simulink model "quad_SMC"  (R2021a)
settings: Solver=ode3  StartTime=0.0  StopTime=30  FixedStep=0.01  RelTol=1e-3  EnableMultiTasking=on
values from neighbouring files (symbols this model uses):
  g = 9.8    [init_landing.m]
  m = 0.486    [init_landing.m]
undefined symbols (not defined in the file or in its folder): attitude_control, model, position_control, sigbuilder_block, sliding_var
libraries: simulink x7, fuzblock x6, eeGeneralControl x3
settings Model: Creator=smishra  LastModifiedBy=fairu
settings SolverCC: AlgebraicLoopSolver=TrustRegion
settings DataIOCC: LimitDataPoints=on  SaveFormat=Array  ReturnWorkspaceOutputs=off  Refine=5
settings OptimizationCC: LifeSpan=inf
settings DebuggingCC: SFUnexpectedBacktrackingDiag=warning  SFNoUnconditionalDefaultTransitionDiag=warning  SFExecutionAtInitializationDiag=none  SFMachineParentedDataDiag=warning  ArithmeticOperatorsInVariantConditions=warning
settings HardwareCC: ProdBitPerPointer=32  ProdBitPerSizeT=32  ProdBitPerPtrDiffT=32  ProdLargestAtomicFloat=None  ProdIntDivRoundTo=Undefined  ProdEndianess=Unspecified  ProdWordSize=32  ProdHWDeviceType=32-bit Generic
settings ModelReferenceCC: PropagateSignalLabelsOutOfModel=off
settings SFSimCC: SimUseLocalCustomCode=off  CustomCodeUndefinedFunction=UseInterfaceOnly
settings RTWCC: RTWUseLocalCustomCode=off
settings CodeAppCC: StateflowObjectComments=on
settings GRTTargetCC: TargetLangStandard=C89/C90 (ANSI)
settings ConfigComp: CovMetricSettings=dw  CovSaveCumulativeToWorkspaceVar=on  CovSaveSingleToWorkspaceVar=on  CovExternalEMLEnable=off

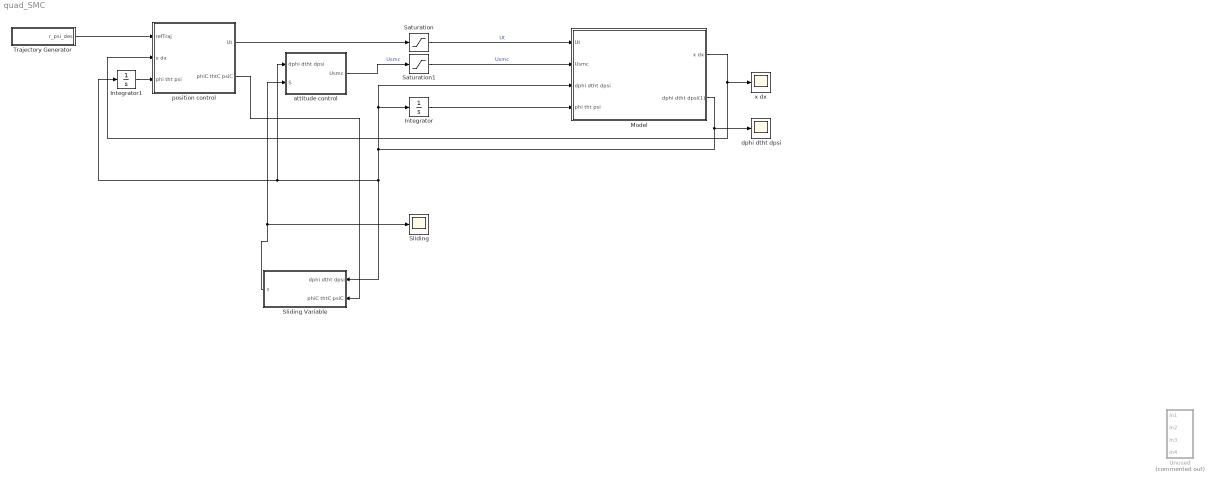
== system quad_SMC ==
  Integrator : Integrator
  Integrator1 : Integrator
  Model : Subsystem
  Saturation : Saturate  UpperLimit=2*m*g  LowerLimit=0
  Saturation1 : Saturate  UpperLimit=0.2  LowerLimit=-0.2
  Sliding : Scope
  Sliding Variable : Subsystem
  Trajectory Generator : Subsystem
  Unused : Subsystem  Commented=on
  attitude control : Subsystem
  dphi dtht dpsi : Scope
  position control : Subsystem
  x dx : Scope
  wires:
  Trajectory Generator/1(r_psi_des) -> position control/1(refTraj)
  Model/2(dphi dtht dpsi(1)) -> dphi dtht dpsi/1, Integrator1/1, attitude control/1(dphi dtht dpsi), Sliding Variable/1(dphi dtht dpsi), Integrator/1, Model/3(dphi dtht dpsi)
  Integrator/1 -> Model/4(phi tht psi)
  Integrator1/1 -> position control/3(phi tht psi)
  Model/1(x dx) -> x dx/1, position control/2(x dx)
  Sliding Variable/1(s) -> attitude control/2(S), Sliding/1
  position control/2(phiC thtC psiC) -> Sliding Variable/2(phiC thtC psiC)
  Saturation/1 -> Model/1(Ut)  "Ut"
  position control/1(Ut) -> Saturation/1
  attitude control/1(Usmc) -> Saturation1/1  "Usmc"
  Saturation1/1 -> Model/2(Usmc)  "Usmc"

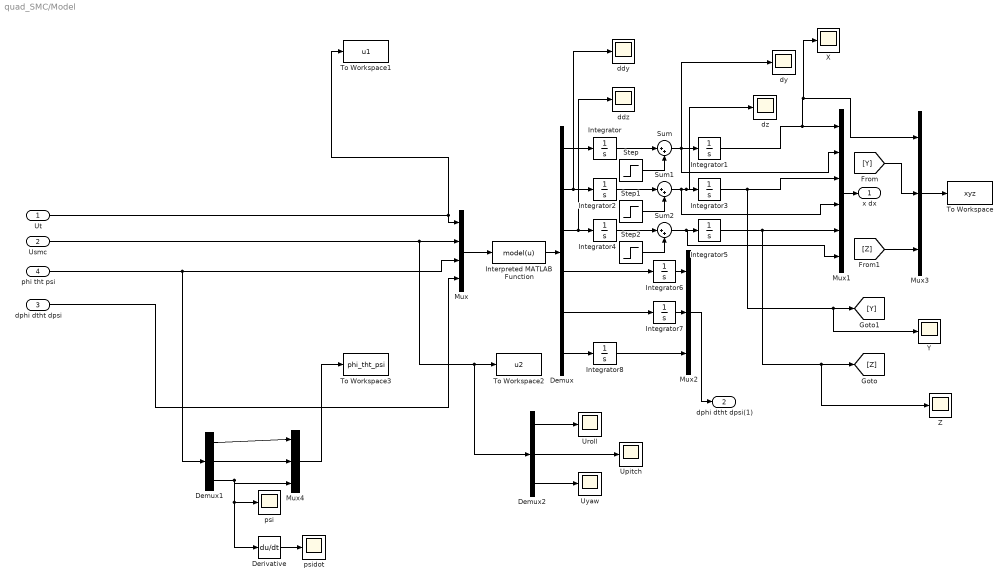
== system quad_SMC/Model ==
  Ut : Inport
  Usmc : Inport  Port=2
  dphi dtht dpsi : Inport  Port=3
  phi tht psi : Inport  Port=4
  Demux : Demux  Outputs=6
  Demux1 : Demux  Outputs=3
  Demux2 : Demux  Outputs=3
  Derivative : Derivative
  Integrator{,1..2,4..8} (8 alike) : Integrator
  Integrator3 : Integrator  InitialCondition=8
  Interpreted MATLAB Function : MATLABFcn  MATLABFcn=model(u)  OutputDimensions=6
  Mux : Mux
  Mux1 : Mux  Inputs=6
  Mux2 : Mux  Inputs=3
  Mux3 : Mux  Inputs=3
  Mux4 : Mux  Inputs=3
  Step : Step  Time=25  After=5  SampleTime=0
  Step1 : Step  Time=25  After=5  SampleTime=0
  Step2 : Step  Time=25  After=5  SampleTime=0
  Sum : Sum  Inputs=|++
  Sum1 : Sum  Inputs=|++
  Sum2 : Sum  Inputs=|++
  To Workspace : ToWorkspace  VariableName=xyz  SampleTime=-1
  To Workspace1 : ToWorkspace  VariableName=u1  SampleTime=-1
  To Workspace2 : ToWorkspace  VariableName=u2  SampleTime=-1
  To Workspace3 : ToWorkspace  VariableName=phi_tht_psi  SampleTime=-1
  Upitch : Scope
  Uroll : Scope
  Uyaw : Scope
  X : Scope
  Y : Scope
  Z : Scope
  ddy : Scope
  ddz : Scope
  dy : Scope
  dz : Scope
  psi : Scope
  psidot : Scope
  x dx : Outport
  dphi dtht dpsi(1) : Outport  Port=2
  wires:
  Mux2/1 -> dphi dtht dpsi(1)/1
  Mux1/1 -> x dx/1
  Mux/1 -> Interpreted MATLAB Function/1
  Integrator3/1 -> Mux1/3, Y/1, [Y]
  Demux/3 -> ddz/1, Integrator4/1
  Demux/1 -> Integrator/1
  Integrator1/1 -> X/1, Mux3/1, Mux1/1
  Integrator7/1 -> Mux2/2
  Interpreted MATLAB Function/1 -> Demux/1
  Integrator8/1 -> Mux2/3
  Demux/2 -> ddy/1, Integrator2/1
  Integrator6/1 -> Mux2/1
  phi tht psi/1 -> Demux1/1, Mux/3
  Mux3/1 -> To Workspace/1
  Ut/1 -> Mux/1, To Workspace1/1
  Usmc/1 -> Mux/2, Demux2/1, To Workspace2/1
  dphi dtht dpsi/1 -> Mux/4
  Demux/4 -> Integrator6/1
  Demux/5 -> Integrator7/1
  Demux/6 -> Integrator8/1
  Integrator/1 -> Sum/1
  Sum/1 -> dy/1, Mux1/2, Integrator1/1
  Integrator2/1 -> Sum1/1
  Sum1/1 -> Mux1/4, dz/1, Integrator3/1
  Integrator4/1 -> Sum2/1
  Step/1 -> Sum/2
  Step1/1 -> Sum1/2
  Step2/1 -> Sum2/2
  Sum2/1 -> Mux1/6, Integrator5/1
  Integrator5/1 -> Z/1, [Z], Mux1/5
  [Y] -> Mux3/2
  [Z] -> Mux3/3
  Demux1/1 -> Mux4/1
  Demux1/2 -> Mux4/2
  Demux1/3 -> Derivative/1, psi/1, Mux4/3
  Mux4/1 -> To Workspace3/1
  Derivative/1 -> psidot/1
  Demux2/1 -> Uroll/1
  Demux2/2 -> Upitch/1
  Demux2/3 -> Uyaw/1

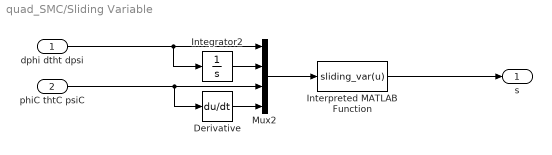
== system quad_SMC/Sliding Variable ==
  dphi dtht dpsi : Inport
  phiC thtC psiC : Inport  Port=2
  Derivative : Derivative
  Integrator2 : Integrator
  Interpreted MATLAB Function : MATLABFcn  MATLABFcn=sliding_var(u)  OutputDimensions=3
  Mux2 : Mux
  s : Outport
  wires:
  Integrator2/1 -> Mux2/2
  Mux2/1 -> Interpreted MATLAB Function/1
  dphi dtht dpsi/1 -> Integrator2/1, Mux2/1
  Interpreted MATLAB Function/1 -> s/1
  phiC thtC psiC/1 -> Derivative/1, Mux2/3
  Derivative/1 -> Mux2/4

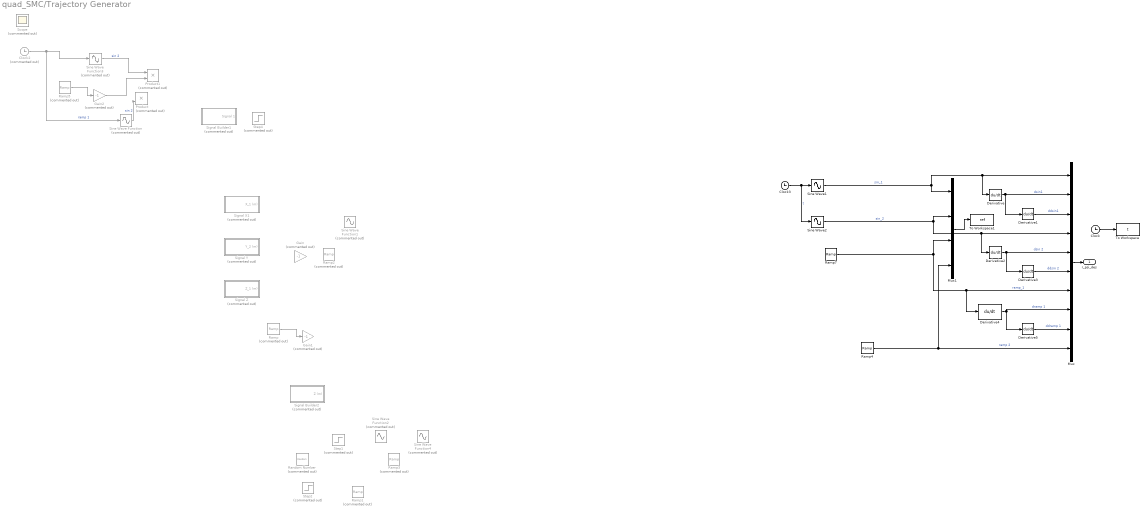
== system quad_SMC/Trajectory Generator ==
  Clock : Clock
  Clock2 : Clock  Commented=on
  Clock3 : Clock
  Derivative{,1..5} (6 alike) : Derivative
  Gain : Gain  Commented=on  Gain=-1
  Gain1 : Gain  Commented=on  Gain=-1
  Gain2 : Gain  Commented=on  Gain=-1
  Mux : Mux  Inputs=10
  Mux1 : Mux
  Product : Product  Commented=on
  Product1 : Product  Commented=on
  Ramp : simulink/Sources/Ramp  Commented=on  slope=1  start=0  InitialOutput=0
  Ramp1 : simulink/Sources/Ramp  Commented=on  slope=0  start=0  InitialOutput=0
  Ramp2 : simulink/Sources/Ramp  Commented=on  slope=0.2  start=0  InitialOutput=-10
  Ramp3 : simulink/Sources/Ramp  Commented=on  slope=0.2  start=0  InitialOutput=-8
  Ramp4 : simulink/Sources/Ramp  slope=0  start=0  InitialOutput=0
  Ramp5 : simulink/Sources/Ramp  Commented=on  slope=1  start=0  InitialOutput=0
  Ramp7 : simulink/Sources/Ramp  slope=0.2  start=0  InitialOutput=0
  Random Number : RandomNumber  Commented=on  SampleTime=0
  Scope : Scope  Commented=on
  Signal Builder1 : Subsystem  Tag=STV Subsys  Commented=on  LoadFcn=sigbuilder_block('load');  StartFcn=sigbuilder_block('start');  StopFcn=sigbuilder_block('stop');  ClipboardFcn=sigbuilder_block('clipboard');  mask(Sigbuilder block){tuvar=[0:10]}
      mask help: Simulink:masks:SigbuilderBlock_MD
      mask init:
      | if ~strcmp(get_param(bdroot(gcbh),'SimulationStatus'),'stopped') tuvar = sigbuilder_block('maskInit'); end
      settings: CopyFcn=sigbuilder_block('copy');  DeleteFcn=sigbuilder_block('delete');  ModelCloseFcn=sigbuilder_block('modelClose');  PreSaveFcn=sigbuilder_block('preSave');  PauseFcn=sigbuilder_block('pause');  ContinueFcn=sigbuilder_block('continue');  NameChangeFcn=sigbuilder_block('namechange');  OpenFcn=sigbuilder_block('open',[411 128.5 543.5 351.5 ]);  CloseFcn=sigbuilder_block('close');
      mask Display: plot(0, 0, 100, 100,[2, 2, 32, 32, 2], [68, 8, 8, 68, 68],[32, 2], [38, 38], [32, 19, 2],[53, 60, 44], [32, 17, 17, 2],[16, 16, 31, 31]);txt = getActiveGroup(gcbh);text(2, 100, txt,'verticalAlignment', 'top');
  Signal Builder2 : Subsystem  Tag=STV Subsys  Commented=on  LoadFcn=sigbuilder_block('load');  StartFcn=sigbuilder_block('start');  StopFcn=sigbuilder_block('stop');  ClipboardFcn=sigbuilder_block('clipboard');  mask(Sigbuilder block){tuvar=[0:10]}
      mask help: Simulink:masks:SigbuilderBlock_MD
      mask init:
      | if ~strcmp(get_param(bdroot(gcbh),'SimulationStatus'),'stopped') tuvar = sigbuilder_block('maskInit'); end
      settings: CopyFcn=sigbuilder_block('copy');  DeleteFcn=sigbuilder_block('delete');  ModelCloseFcn=sigbuilder_block('modelClose');  PreSaveFcn=sigbuilder_block('preSave');  PauseFcn=sigbuilder_block('pause');  ContinueFcn=sigbuilder_block('continue');  NameChangeFcn=sigbuilder_block('namechange');  OpenFcn=sigbuilder_block('open',[5.5 30 949 418 ]);  CloseFcn=sigbuilder_block('close');
      mask Display: plot(0, 0, 100, 100,[2, 2, 32, 32, 2], [68, 8, 8, 68, 68],[32, 2], [38, 38], [32, 19, 2],[53, 60, 44], [32, 17, 17, 2],[16, 16, 31, 31]);txt = getActiveGroup(gcbh);text(2, 100, txt,'verticalAlignment', 'top');
  Signal X1 : Subsystem  Tag=STV Subsys  Commented=on  LoadFcn=sigbuilder_block('load');  StartFcn=sigbuilder_block('start');  StopFcn=sigbuilder_block('stop');  ClipboardFcn=sigbuilder_block('clipboard');  mask(Sigbuilder block){tuvar=[0:10]}
      mask help: Simulink:masks:SigbuilderBlock_MD
      mask init:
      | if ~strcmp(get_param(bdroot(gcbh),'SimulationStatus'),'stopped') tuvar = sigbuilder_block('maskInit'); end
      settings: CopyFcn=sigbuilder_block('copy');  DeleteFcn=sigbuilder_block('delete');  ModelCloseFcn=sigbuilder_block('modelClose');  PreSaveFcn=sigbuilder_block('preSave');  PauseFcn=sigbuilder_block('pause');  ContinueFcn=sigbuilder_block('continue');  NameChangeFcn=sigbuilder_block('namechange');  OpenFcn=sigbuilder_block('open',[411 128.5 543.5 351.5 ]);  CloseFcn=sigbuilder_block('close');
      mask Display: plot(0, 0, 100, 100,[2, 2, 32, 32, 2], [68, 8, 8, 68, 68],[32, 2], [38, 38], [32, 19, 2],[53, 60, 44], [32, 17, 17, 2],[16, 16, 31, 31]);txt = getActiveGroup(gcbh);text(2, 100, txt,'verticalAlignment', 'top');
  Signal Y : Subsystem  Tag=STV Subsys  Commented=on  LoadFcn=sigbuilder_block('load');  StartFcn=sigbuilder_block('start');  StopFcn=sigbuilder_block('stop');  ClipboardFcn=sigbuilder_block('clipboard');  mask(Sigbuilder block){tuvar=[0:10]}
      mask help: Simulink:masks:SigbuilderBlock_MD
      mask init:
      | if ~strcmp(get_param(bdroot(gcbh),'SimulationStatus'),'stopped') tuvar = sigbuilder_block('maskInit'); end
      settings: CopyFcn=sigbuilder_block('copy');  DeleteFcn=sigbuilder_block('delete');  ModelCloseFcn=sigbuilder_block('modelClose');  PreSaveFcn=sigbuilder_block('preSave');  PauseFcn=sigbuilder_block('pause');  ContinueFcn=sigbuilder_block('continue');  NameChangeFcn=sigbuilder_block('namechange');  OpenFcn=sigbuilder_block('open',[411 128.5 543.5 351.5 ]);  CloseFcn=sigbuilder_block('close');
      mask Display: plot(0, 0, 100, 100,[2, 2, 32, 32, 2], [68, 8, 8, 68, 68],[32, 2], [38, 38], [32, 19, 2],[53, 60, 44], [32, 17, 17, 2],[16, 16, 31, 31]);txt = getActiveGroup(gcbh);text(2, 100, txt,'verticalAlignment', 'top');
  Signal Z : Subsystem  Tag=STV Subsys  Commented=on  LoadFcn=sigbuilder_block('load');  StartFcn=sigbuilder_block('start');  StopFcn=sigbuilder_block('stop');  ClipboardFcn=sigbuilder_block('clipboard');  mask(Sigbuilder block){tuvar=[0:10]}
      mask help: Simulink:masks:SigbuilderBlock_MD
      mask init:
      | if ~strcmp(get_param(bdroot(gcbh),'SimulationStatus'),'stopped') tuvar = sigbuilder_block('maskInit'); end
      settings: CopyFcn=sigbuilder_block('copy');  DeleteFcn=sigbuilder_block('delete');  ModelCloseFcn=sigbuilder_block('modelClose');  PreSaveFcn=sigbuilder_block('preSave');  PauseFcn=sigbuilder_block('pause');  ContinueFcn=sigbuilder_block('continue');  NameChangeFcn=sigbuilder_block('namechange');  OpenFcn=sigbuilder_block('open',[411 128.5 543.5 351.5 ]);  CloseFcn=sigbuilder_block('close');
      mask Display: plot(0, 0, 100, 100,[2, 2, 32, 32, 2], [68, 8, 8, 68, 68],[32, 2], [38, 38], [32, 19, 2],[53, 60, 44], [32, 17, 17, 2],[16, 16, 31, 31]);txt = getActiveGroup(gcbh);text(2, 100, txt,'verticalAlignment', 'top');
  Sine Wave Function : Sin  Commented=on  TimeSource=Use external signal  Amplitude=10  Frequency=0.1  Phase=pi/2  SampleTime=0
  Sine Wave Function1 : Sin  Commented=on  TimeSource=Use external signal  Amplitude=8  Frequency=0.1  Phase=pi/2  SampleTime=0
  Sine Wave Function2 : Sin  Commented=on  TimeSource=Use external signal  Amplitude=10  Frequency=0.1  SampleTime=0
  Sine Wave Function3 : Sin  Commented=on  TimeSource=Use external signal  Amplitude=10  Frequency=0.1  SampleTime=0
  Sine Wave Function4 : Sin  Commented=on  TimeSource=Use external signal  Amplitude=10  Frequency=0.1  Phase=pi/2  SampleTime=0
  Sine Wave1 : Sin  TimeSource=Use external signal  Amplitude=8  Frequency=0.1  SampleTime=0
  Sine Wave2 : Sin  TimeSource=Use external signal  Amplitude=8  Frequency=0.1  Phase=pi/2  SampleTime=0
  Step1 : Step  Commented=on  Before=-8  SampleTime=0
  Step2 : Step  Commented=on  SampleTime=0
  Step4 : Step  Commented=on  After=8  SampleTime=0
  To Workspace : ToWorkspace  VariableName=t  SampleTime=-1
  To Workspace1 : ToWorkspace  VariableName=ref  SampleTime=-1
  r_psi_des : Outport
  wires:
  Derivative2/1 -> Mux/5, Derivative3/1  "dsin 2"
  Derivative4/1 -> Mux/8, Derivative5/1  "dramp 1"
  Derivative/1 -> Mux/2, Derivative1/1  "dsin1"
  Derivative1/1 -> Mux/3  "ddsin1"
  Derivative3/1 -> Mux/6  "ddsin 2"
  Derivative5/1 -> Mux/9  "ddramp 1"
  Ramp4/1 -> Mux1/4, Mux/10  "ramp 2"
  Mux/1 -> r_psi_des/1
  Clock/1 -> To Workspace/1
  Mux1/1 -> To Workspace1/1
  Sine Wave1/1 -> Mux/1, Derivative/1, Mux1/1  "sin_1"
  Ramp/1 -> Gain1/1
  Sine Wave Function/1 -> Product/2  "sin 2"
  Clock2/1 -> Sine Wave Function/1, Sine Wave Function3/1  "ramp 1"
  Ramp5/1 -> Gain2/1
  Gain2/1 -> Product1/2
  Sine Wave Function3/1 -> Product1/1  "sin 2"
  Ramp7/1 -> Derivative4/1, Mux/7, Mux1/3  "ramp_1"
  Sine Wave2/1 -> Mux1/2, Derivative2/1, Mux/4  "sin_2"
  Clock3/1 -> Sine Wave2/1, Sine Wave1/1  "t"

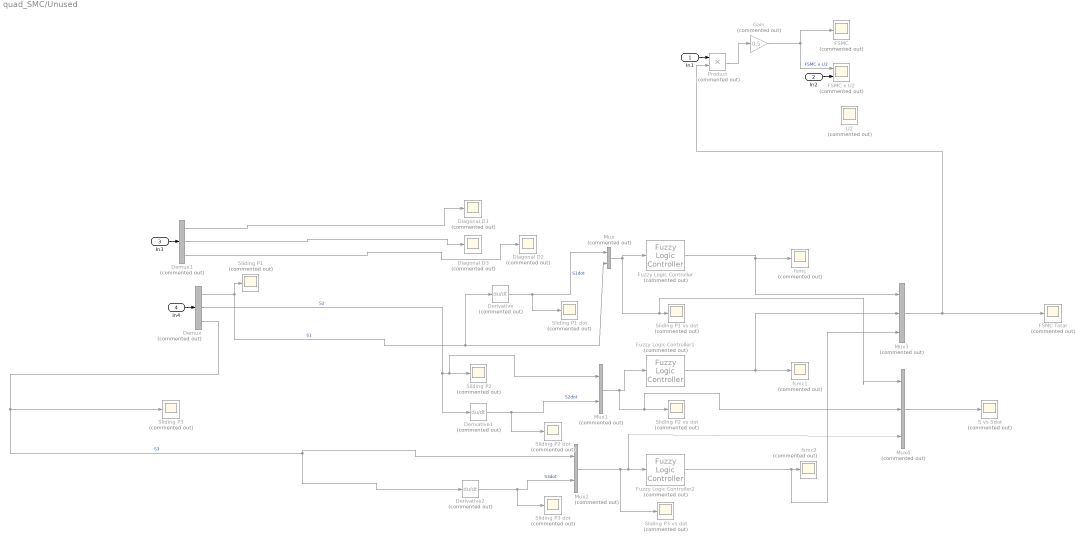
== system quad_SMC/Unused ==
  In1 : Inport
  In2 : Inport  Port=2
  In3 : Inport  Port=3
  In4 : Inport  Port=4
  Demux : Demux  Commented=on  Outputs=3
  Demux1 : Demux  Commented=on  Outputs=3
  Derivative : Derivative  Commented=on
  Derivative1 : Derivative  Commented=on
  Derivative2 : Derivative  Commented=on
  Diagonal D1 : Scope  Commented=on
  Diagonal D2 : Scope  Commented=on
  Diagonal D3 : Scope  Commented=on
  FSMC : Scope  Commented=on
  FSMC Total : Scope  Commented=on
  FSMC x U2 : Scope  Commented=on  NumInputPorts=2
  Fuzzy Logic Controller : fuzblock/Fuzzy Logic  Controller  Commented=on  FIS='smc.fis'  OutputSampleNumber=101  DataType=double  FuzzifiedInputs=off  RuleFiringStrengths=off  RuleOutputs=off  AggregatedOutputs=off  SimulateUsing=Interpreted execution  OutOfRangeInputValueMessage=warning  NoRuleFiredMessage=warning  EmptyOutputFuzzySetMessage=warning
  Fuzzy Logic Controller1 : fuzblock/Fuzzy Logic  Controller  Commented=on  FIS='smc_21.fis'  OutputSampleNumber=101  DataType=double  FuzzifiedInputs=off  RuleFiringStrengths=off  RuleOutputs=off  AggregatedOutputs=off  SimulateUsing=Interpreted execution  OutOfRangeInputValueMessage=warning  NoRuleFiredMessage=warning  EmptyOutputFuzzySetMessage=warning
  Fuzzy Logic Controller2 : fuzblock/Fuzzy Logic  Controller  Commented=on  FIS='smc_31.fis'  OutputSampleNumber=101  DataType=double  FuzzifiedInputs=off  RuleFiringStrengths=off  RuleOutputs=off  AggregatedOutputs=off  SimulateUsing=Interpreted execution  OutOfRangeInputValueMessage=warning  NoRuleFiredMessage=warning  EmptyOutputFuzzySetMessage=warning
  Gain : Gain  Commented=on  Gain=0.5
  Mux : Mux  Commented=on  Inputs=2
  Mux1 : Mux  Commented=on  Inputs=2
  Mux2 : Mux  Commented=on  Inputs=2
  Mux3 : Mux  Commented=on  Inputs=3
  Mux4 : Mux  Commented=on  Inputs=3
  Product : Product  Commented=on
  S vs Sdot : Scope  Commented=on
  Sliding P1 : Scope  Commented=on
  Sliding P1 dot : Scope  Commented=on
  Sliding P1 vs dot : Scope  Commented=on
  Sliding P2 : Scope  Commented=on
  Sliding P2 dot : Scope  Commented=on
  Sliding P2 vs dot : Scope  Commented=on
  Sliding P3 : Scope  Commented=on
  Sliding P3 dot : Scope  Commented=on
  Sliding P3 vs dot : Scope  Commented=on
  U2 : Scope  Commented=on
  fsmc : Scope  Commented=on
  fsmc1 : Scope  Commented=on
  fsmc2 : Scope  Commented=on
  wires:
  Product/1 -> Gain/1
  Demux/3 -> Derivative2/1, Mux2/1, Sliding P3/1  "S3"
  In2/1 -> FSMC x U2/2
  Fuzzy Logic Controller/1 -> Mux3/1, fsmc/1
  Mux1/1 -> Mux4/2, Sliding P2 vs dot/1, Fuzzy Logic Controller1/1
  In4/1 -> Demux/1
  Demux1/3 -> Diagonal D2/1
  Mux/1 -> Mux4/1, Sliding P1 vs dot/1, Fuzzy Logic Controller/1
  Demux/2 -> Derivative1/1, Mux1/1, Sliding P2/1  "S2"
  Fuzzy Logic Controller1/1 -> Mux3/2, fsmc1/1
  Derivative/1 -> Sliding P1 dot/1, Mux/1  "S1dot"
  Mux3/1 -> Product/2, FSMC Total/1
  Fuzzy Logic Controller2/1 -> Mux3/3, fsmc2/1
  Demux1/2 -> Diagonal D3/1
  Demux/1 -> Sliding P1/1, Derivative/1, Mux/2  "S1"
  Derivative2/1 -> Sliding P3 dot/1, Mux2/2  "S3dot"
  Mux4/1 -> S vs Sdot/1
  Derivative1/1 -> Sliding P2 dot/1, Mux1/2  "S2dot"
  Gain/1 -> FSMC/1, FSMC x U2/1  "FSMC x U2"
  Demux1/1 -> Diagonal D1/1
  In3/1 -> Demux1/1
  Mux2/1 -> Sliding P3 vs dot/1, Mux4/3, Fuzzy Logic Controller2/1
  In1/1 -> Product/1

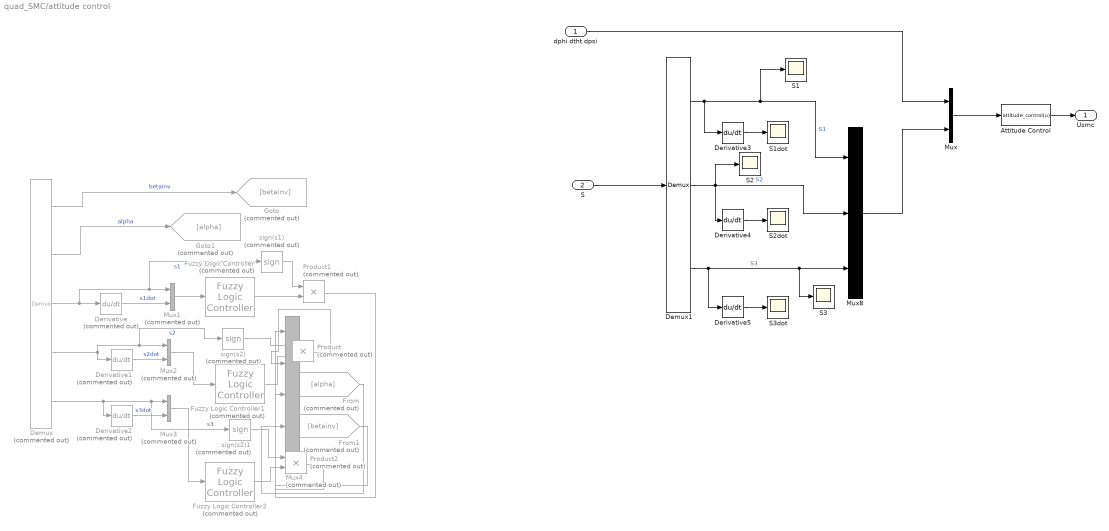
== system quad_SMC/attitude control ==
  dphi dtht dpsi : Inport
  S : Inport  Port=2
  Attitude Control : MATLABFcn  MATLABFcn=attitude_control(u)  OutputDimensions=3
  Demux : Demux  Commented=on  Outputs=5
  Demux1 : Demux  Outputs=3
  Derivative : Derivative  Commented=on
  Derivative1 : Derivative  Commented=on
  Derivative2 : Derivative  Commented=on
  Derivative3 : Derivative
  Derivative4 : Derivative
  Derivative5 : Derivative
  From : From  Commented=on  GotoTag=alpha
  From1 : From  Commented=on  GotoTag=betainv
  Fuzzy Logic Controller : fuzblock/Fuzzy Logic  Controller  Commented=on  FIS='smc.fis'  OutputSampleNumber=101  DataType=double  FuzzifiedInputs=off  RuleFiringStrengths=off  RuleOutputs=off  AggregatedOutputs=off  SimulateUsing=Interpreted execution  OutOfRangeInputValueMessage=warning  NoRuleFiredMessage=warning  EmptyOutputFuzzySetMessage=warning
  Fuzzy Logic Controller1 : fuzblock/Fuzzy Logic  Controller  Commented=on  FIS='tipper.fis'  OutputSampleNumber=101  DataType=double  FuzzifiedInputs=off  RuleFiringStrengths=off  RuleOutputs=off  AggregatedOutputs=off  SimulateUsing=Interpreted execution  OutOfRangeInputValueMessage=warning  NoRuleFiredMessage=warning  EmptyOutputFuzzySetMessage=warning
  Fuzzy Logic Controller2 : fuzblock/Fuzzy Logic  Controller  Commented=on  FIS='tipper.fis'  OutputSampleNumber=101  DataType=double  FuzzifiedInputs=off  RuleFiringStrengths=off  RuleOutputs=off  AggregatedOutputs=off  SimulateUsing=Interpreted execution  OutOfRangeInputValueMessage=warning  NoRuleFiredMessage=warning  EmptyOutputFuzzySetMessage=warning
  Goto : Goto  Commented=on  GotoTag=betainv
  Goto1 : Goto  Commented=on  GotoTag=alpha
  Mux : Mux  Inputs=2
  Mux1 : Mux  Commented=on  Inputs=2
  Mux2 : Mux  Commented=on  Inputs=2
  Mux3 : Mux  Commented=on  Inputs=2
  Mux4 : Mux  Commented=on  Inputs=5
  Mux8 : Mux  Inputs=3
  Product : Product  Commented=on
  Product1 : Product  Commented=on
  Product2 : Product  Commented=on
  S1 : Scope
  S1dot : Scope
  S2 : Scope
  S2dot : Scope
  S3 : Scope
  S3dot : Scope
  sign(s1) : Signum  Commented=on
  sign(s2) : Signum  Commented=on
  sign(s2)1 : Signum  Commented=on
  Usmc : Outport
  wires:
  Mux/1 -> Attitude Control/1
  dphi dtht dpsi/1 -> Mux/1
  S/1 -> Demux1/1
  Mux1/1 -> Fuzzy Logic Controller/1
  Demux/3 -> sign(s1)/1, Mux1/1, Derivative/1  "s1"
  Derivative/1 -> Mux1/2  "s1dot"
  Demux/4 -> Derivative1/1, sign(s2)/1, Mux2/1  "s2"
  Mux2/1 -> Fuzzy Logic Controller1/1
  Derivative1/1 -> Mux2/2  "s2dot"
  Demux/5 -> Derivative2/1, sign(s2)1/1, Mux3/1  "s3"
  Mux3/1 -> Fuzzy Logic Controller2/1
  Fuzzy Logic Controller1/1 -> Product/2
  Demux/1 -> Goto/1  "betainv"
  Demux/2 -> Goto1/1  "alpha"
  Attitude Control/1 -> Usmc/1
  Derivative2/1 -> Mux3/2  "s3dot"
  Product/1 -> Mux4/2
  sign(s2)/1 -> Product/1
  sign(s1)/1 -> Product1/1
  Fuzzy Logic Controller/1 -> Product1/2
  Product1/1 -> Mux4/1
  sign(s2)1/1 -> Product2/1
  Fuzzy Logic Controller2/1 -> Product2/2
  Product2/1 -> Mux4/3
  From/1 -> Mux4/4
  From1/1 -> Mux4/5
  Demux1/1 -> Derivative3/1, S1/1, Mux8/1  "S1"
  Demux1/2 -> S2/1, Derivative4/1, Mux8/2  "S2"
  Demux1/3 -> Derivative5/1, S3/1, Mux8/3  "S3"
  Mux8/1 -> Mux/2
  Derivative3/1 -> S1dot/1
  Derivative4/1 -> S2dot/1
  Derivative5/1 -> S3dot/1

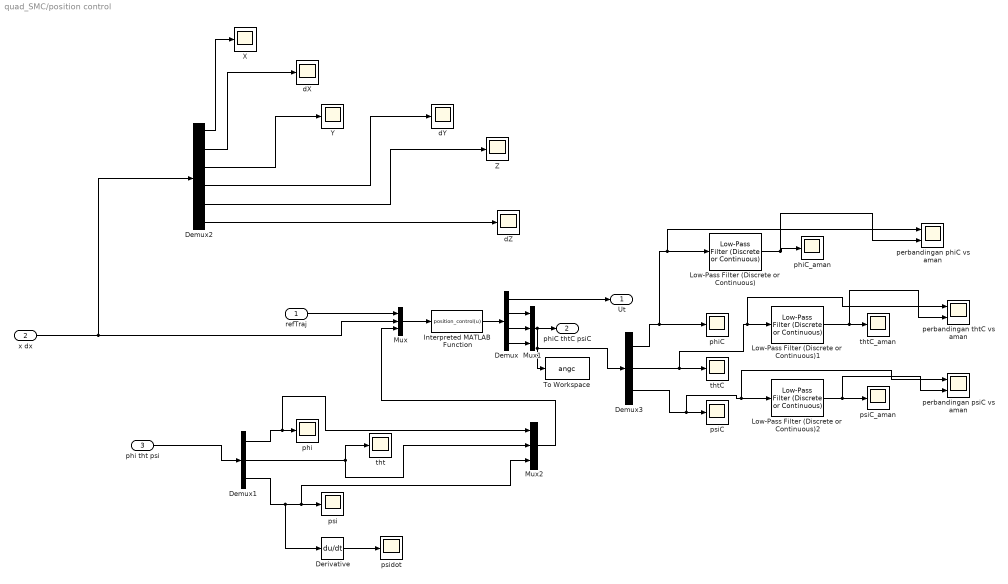
== system quad_SMC/position control ==
  refTraj : Inport
  x dx : Inport  Port=2
  phi tht psi : Inport  Port=3
  Demux : Demux
  Demux1 : Demux  Outputs=3
  Demux2 : Demux  Outputs=6
  Demux3 : Demux  Outputs=3
  Derivative : Derivative
  Interpreted MATLAB Function : MATLABFcn  MATLABFcn=position_control(u)  OutputDimensions=4
  Low-Pass Filter (Discrete or Continuous) : eeGeneralControl/Low-Pass Filter (Discrete or Continuous)  K=1  T=1  B=inf  A=-inf  init_option=Inherited from block input  x0=0  Ts=-1
  Low-Pass Filter (Discrete or Continuous)1 : eeGeneralControl/Low-Pass Filter (Discrete or Continuous)  K=1  T=1  B=inf  A=-inf  init_option=Inherited from block input  x0=0  Ts=-1
  Low-Pass Filter (Discrete or Continuous)2 : eeGeneralControl/Low-Pass Filter (Discrete or Continuous)  K=1  T=1  B=inf  A=-inf  init_option=Inherited from block input  x0=0  Ts=-1
  Mux : Mux  Inputs=3
  Mux1 : Mux  Inputs=3
  Mux2 : Mux  Inputs=3
  To Workspace : ToWorkspace  VariableName=angc  SampleTime=-1
  X : Scope
  Y : Scope
  Z : Scope
  dX : Scope
  dY : Scope
  dZ : Scope
  perbandingan phiC vs aman : Scope  NumInputPorts=2
  perbandingan psiC vs aman : Scope  NumInputPorts=2
  perbandingan thtC vs aman : Scope  NumInputPorts=2
  phi : Scope
  phiC : Scope
  phiC_aman : Scope
  psi : Scope
  psiC : Scope
  psiC_aman : Scope
  psidot : Scope
  tht : Scope
  thtC : Scope
  thtC_aman : Scope
  Ut : Outport
  phiC thtC psiC : Outport  Port=2
  wires:
  Mux/1 -> Interpreted MATLAB Function/1
  refTraj/1 -> Mux/1
  x dx/1 -> Demux2/1, Mux/2
  phi tht psi/1 -> Demux1/1
  Interpreted MATLAB Function/1 -> Demux/1
  Demux/1 -> Ut/1
  Demux/2 -> Mux1/1
  Demux/3 -> Mux1/2
  Demux/4 -> Mux1/3
  Mux1/1 -> Demux3/1, To Workspace/1, phiC thtC psiC/1
  Demux1/1 -> Mux2/1, phi/1
  Demux1/2 -> tht/1, Mux2/2
  Derivative/1 -> psidot/1
  Demux1/3 -> Derivative/1, Mux2/3, psi/1
  Mux2/1 -> Mux/3
  Demux2/2 -> dX/1
  Demux2/1 -> X/1
  Demux2/3 -> Y/1
  Demux2/4 -> dY/1
  Demux2/5 -> Z/1
  Demux2/6 -> dZ/1
  Demux3/1 -> perbandingan phiC vs aman/1, Low-Pass Filter (Discrete or Continuous)/1, phiC/1
  Demux3/2 -> perbandingan thtC vs aman/1, Low-Pass Filter (Discrete or Continuous)1/1, thtC/1
  Demux3/3 -> perbandingan psiC vs aman/1, Low-Pass Filter (Discrete or Continuous)2/1, psiC/1
  Low-Pass Filter (Discrete or Continuous)/1 -> perbandingan phiC vs aman/2, phiC_aman/1
  Low-Pass Filter (Discrete or Continuous)1/1 -> perbandingan thtC vs aman/2, thtC_aman/1
  Low-Pass Filter (Discrete or Continuous)2/1 -> perbandingan psiC vs aman/2, psiC_aman/1

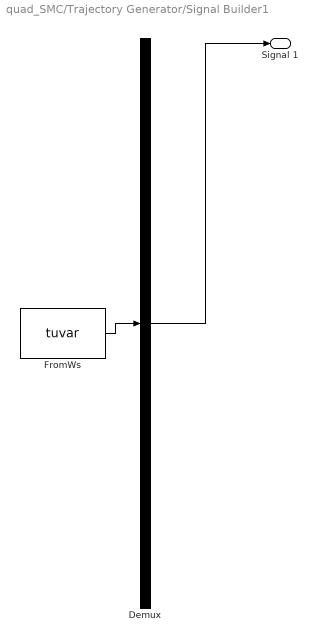
== system quad_SMC/Trajectory Generator/Signal Builder1 ==
  Demux : Demux  Tag=STV Demux  Outputs=1
      settings: DisplayOption=none
  FromWs : FromWorkspace  Tag=STV FromWs  VariableName=tuvar
      SigBuilderData=|
      | common.afterFinalStr = 'Extrapolate'
      | common.sampleTime = 0
      | dataSet.timeRange = [0 10]
      | dataSet.name = 'Group 1'
      | sbobj.Groups.Name = 'Group 1'
      | sbobj.Groups.Signals.Name = 'Signal 1'
      | sbobj.Groups.Signals.XData = [0 1 1 8 8 10]
      | sbobj.Groups.Signals.YData = [-1.48 -1.48 1 1 0 0]
  Signal 1 : Outport  Tag=STV Outport
  wires:
  Demux/1 -> Signal 1/1
  FromWs/1 -> Demux/1

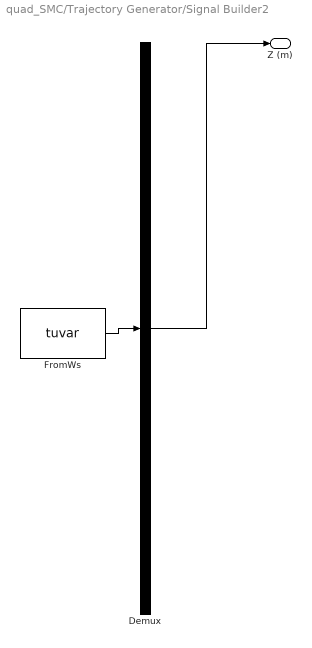
== system quad_SMC/Trajectory Generator/Signal Builder2 ==
  Demux : Demux  Tag=STV Demux  Outputs=1
      settings: DisplayOption=none
  FromWs : FromWorkspace  Tag=STV FromWs  VariableName=tuvar
      SigBuilderData=|
      | common.afterFinalStr = 'Extrapolate'
      | common.sampleTime = 0
      | dataSet.timeRange = [0 100]
      | dataSet.name = 'Sheet1'
      | sbobj.Groups.Name = 'Sheet1'
      | sbobj.Groups.Signals.Name = 'Z (m)'
      | sbobj.Groups.Signals.XData = [0 1 2 3 4 5 6 7 8 9 10 11 12 13 14 15 16 17 18 19 20 21 22 23 24 25 26 27 28 29 30 31 32 33 34 35 36 37 38 39 40 41 42 43 44 45 46 47 48 49 50 51 52 53 54 55 56 57 58 59 60 61 62 63 64 65 66 67 68 69 70 71 72 73 74 75 76 77 78 79 80 81 82 83 84 85 86 87 88 89 90 91 92 93 94 95 96 97 98 99 100]
      | sbobj.Groups.Signals.YData = [10 10 10 10 10 10 10 10 10 10 10 10 10 10 10 10 10 10 10 10 10 10 10 10 10 10 10 10 10 10 10 10 10 10 10 10 10 10 10 10 9 8 7 6 5 4 3 2 1 0.05 0 0 0 0 0 0 0 0 0 0 0 0 0 0 0 0 0 0 0 0 0 0 0 0 0 0 0 0 0 0 0 0 0 0 0 0 0 0 0 0 0 0 0 0 0 0 0 0 0 0 0]
      | sbobj.Groups.TimeRange = [0 100]
  Z (m) : Outport  Tag=STV Outport
  wires:
  Demux/1 -> Z (m)/1
  FromWs/1 -> Demux/1

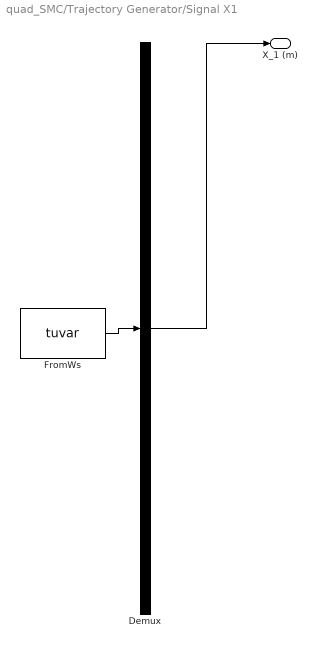
== system quad_SMC/Trajectory Generator/Signal X1 ==
  Demux : Demux  Tag=STV Demux  Outputs=1
      settings: DisplayOption=none
  FromWs : FromWorkspace  Tag=STV FromWs  VariableName=tuvar
      SigBuilderData=|
      | common.afterFinalStr = 'Extrapolate'
      | common.sampleTime = 0
      | dataSet.timeRange = [0 100]
      | dataSet.name = 'Sheet1'
      | sbobj.Groups.Name = 'Sheet1'
      | sbobj.Groups.Signals.Name = 'X_1 (m)'
      | sbobj.Groups.Signals.XData = [0 1 2 3 4 5 6 7 8 9 10 11 12 13 14 15 16 17 18 19 20 21 22 23 24 25 26 26 26.8 28 29 30 31 32 33 34 35 36 37 38 39 40 41 42 43 44 45 46 47 48 49 50 51 52 53 54 55 56 57 58 59 60 61 62 63 64 65 66 67 68 69 70 71 72 73 74 75 76 77 78 79 80 81 82 83 84 85 86 87 88 89 90 91 92 93 94 95 96 97 98 99 100]
      | sbobj.Groups.Signals.YData = [0 0 0 0 0 0 0 0 2 4 6 8 10 10 10 10 8 6 4 2 0 0 0 0 0 0 0 -0.1 -0.1 0 0 0 0 0 0 0 0 0 0 0 0 0 0 0 0 0 0 0 0 0 0 0 0 0 0 0 0 0 0 0 0 0 0 0 0 0 0 0 0 0 0 0 0 0 0 0 0 0 0 0 0 0 0 0 0 0 0 0 0 0 0 0 0 0 0 0 0 0 0 0 0 0]
      | sbobj.Groups.TimeRange = [0 100]
  X_1 (m) : Outport  Tag=STV Outport
  wires:
  Demux/1 -> X_1 (m)/1
  FromWs/1 -> Demux/1

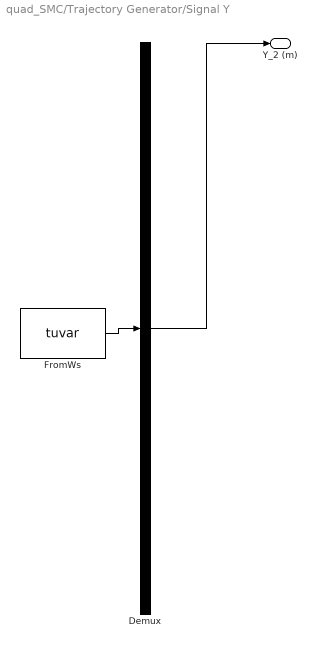
== system quad_SMC/Trajectory Generator/Signal Y ==
  Demux : Demux  Tag=STV Demux  Outputs=1
      settings: DisplayOption=none
  FromWs : FromWorkspace  Tag=STV FromWs  VariableName=tuvar
      SigBuilderData=|
      | common.afterFinalStr = 'Extrapolate'
      | common.sampleTime = 0
      | dataSet.timeRange = [0 100]
      | dataSet.name = 'Sheet1'
      | sbobj.Groups.Name = 'Sheet1'
      | sbobj.Groups.Signals.Name = 'Y_2 (m)'
      | sbobj.Groups.Signals.XData = [0 1 2 3 4 5 6 7 8 9 10 11 12 13 14 15 16 17 18 19 20 21 22 23 24 25 26 27 28 29 30 31 32 33 34 35 36 37 38 39 40 41 42 43 44 45 46 47 48 49 50 51 52 53 54 55 56 57 58 59 60 61 62 63 64 65 66 67 68 69 70 71 72 73 74 75 76 77 78 79 80 81 82 83 84 85 86 87 88 89 90 91 92 93 94 95 96 97 98 99 100]
      | sbobj.Groups.Signals.YData = [0 0 0 0 0 0 0 0 0 0 0 0 2 4 6 8 10 10 10 10 10 10 10 10 10 10 10 10 10 10 10 10 10 10 10 10 10 10 10 10 10 10 10 10 10 10 10 10 10 10 10 10 10 10 10 10 10 10 10 10 10 10 10 10 10 10 10 10 10 10 10 10 10 10 10 10 10 10 10 10 10 10 10 10 10 10 10 10 10 10 10 10 10 10 10 10 10 10 10 10 10]
      | sbobj.Groups.TimeRange = [0 100]
  Y_2 (m) : Outport  Tag=STV Outport
  wires:
  Demux/1 -> Y_2 (m)/1
  FromWs/1 -> Demux/1

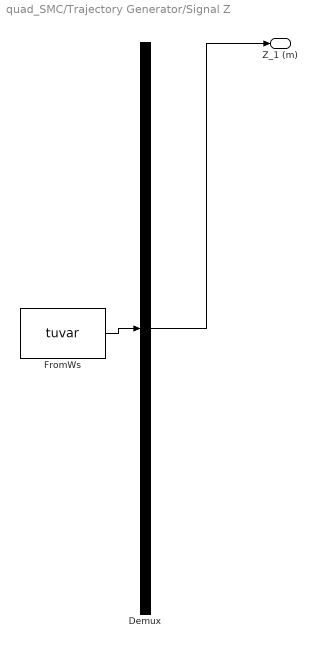
== system quad_SMC/Trajectory Generator/Signal Z ==
  Demux : Demux  Tag=STV Demux  Outputs=1
      settings: DisplayOption=none
  FromWs : FromWorkspace  Tag=STV FromWs  VariableName=tuvar
      SigBuilderData=|
      | common.afterFinalStr = 'Extrapolate'
      | common.sampleTime = 0
      | dataSet.timeRange = [0 100]
      | dataSet.name = 'Sheet1'
      | sbobj.Groups.Name = 'Sheet1'
      | sbobj.Groups.Signals.Name = 'Z_1 (m)'
      | sbobj.Groups.Signals.XData = [0 1 2 3 4 5 6 7 8 9 10 11 12 13 14 15 16 17 18 19 20 21 22 23 24 25 26 27 28 29 100]
      | sbobj.Groups.Signals.YData = [0 0 0 2 4 6 8 10 10 10 10 10 10 10 10 10 10 10 10 10 10 10 10 10 8 6 4 2 0 0 0]
      | sbobj.Groups.TimeRange = [0 100]
  Z_1 (m) : Outport  Tag=STV Outport
  wires:
  Demux/1 -> Z_1 (m)/1
  FromWs/1 -> Demux/1
